simulink model "ResampleUC2Model"  (Simulink 6.6)
settings: Solver=FixedStepDiscrete  StartTime=0.0  StopTime=0  FixedStep=0.1  RelTol=1e-3
libraries: SimITKLibraryUC2 x4, SimITKTransformLibrary2D x1
settings Model: Creator=3kml  LastModifiedBy=3kml

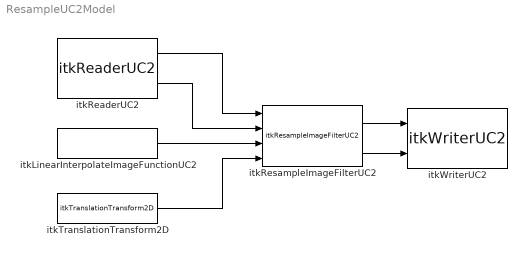
== system ResampleUC2Model ==
  itkLinearInterpolateImageFunctionUC2 : SimITKLibraryUC2/itkLinearInterpolateImageFunctionUC2
  itkReaderUC2 : SimITKLibraryUC2/itkReaderUC2  FileName='cthead1.png'
  itkResampleImageFilterUC2 : SimITKLibraryUC2/itkResampleImageFilterUC2  DefaultPixelValue=0  OutputOrigin=[0 0]  OutputSpacing=[1 1]  Size=[256 256]
  itkTranslationTransform2D : SimITKTransformLibrary2D/itkTranslationTransform2D  Parameters_a=[25 25]  FixedParameters=[]
  itkWriterUC2 : SimITKLibraryUC2/itkWriterUC2  FileName='outputResampleUC2Model.png'
  wires:
  itkReaderUC2/1 -> itkResampleImageFilterUC2/1
  itkReaderUC2/2 -> itkResampleImageFilterUC2/2
  itkResampleImageFilterUC2/1 -> itkWriterUC2/1
  itkResampleImageFilterUC2/2 -> itkWriterUC2/2
  itkLinearInterpolateImageFunctionUC2/1 -> itkResampleImageFilterUC2/3
  itkTranslationTransform2D/1 -> itkResampleImageFilterUC2/4
